simulink model "output_feedback_fixed"  (R2018b)
settings: Solver=VariableStepAuto  StartTime=0.0  StopTime=10  RelTol=1e-3
undefined symbols (not defined in the file): sigbuilder_block
libraries: simulink x1
settings Model: Creator=harkib  LastModifiedBy=Freddy.Kooliyath
settings DebuggingCC: LibraryContextMissingDiagnostic=none
settings SFSimCC: SimUseLocalCustomCode=off
settings RTWCC: RTWUseLocalCustomCode=off

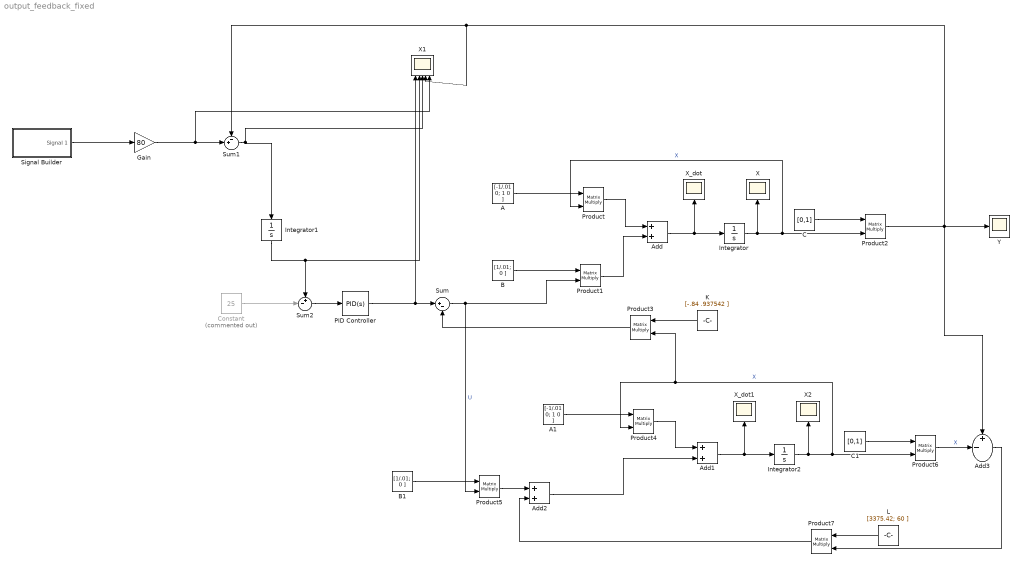
== system output_feedback_fixed ==
  A : Constant  Value=[-1/.01 0; 1 0 ]  VectorParams1D=off
  A1 : Constant  Value=[-1/.01 0; 1 0 ]  VectorParams1D=off
  Add : Sum
  Add1 : Sum
  Add2 : Sum
  Add3 : Sum  Inputs=+-|
  B : Constant  Value=[1/.01; 0 ]  VectorParams1D=off
  B1 : Constant  Value=[1/.01; 0 ]  VectorParams1D=off
  C : Constant  Value=[0,1]  VectorParams1D=off
  C1 : Constant  Value=[0,1]  VectorParams1D=off
  Constant : Constant  Commented=on  Value=25
  Gain : Gain  Gain=80
  Integrator : Integrator
  Integrator1 : Integrator
  Integrator2 : Integrator
  K : Constant  Value=[-.84 .937542 ]  VectorParams1D=off
  L : Constant  Value=[3375.42; 60 ]  VectorParams1D=off
  PID Controller : simulink/Continuous/PID Controller  Controller=PID  Form=Parallel  TimeDomain=Continuous-time  SampleTime=-1  IntegratorMethod=Forward Euler  FilterMethod=Forward Euler  ControllerParametersSource=internal  P=10.0278874654845  I=1.25331489824658  D=2.58452090748358  UseFilter=on  N=1688.62078738213  TunerSelectOption=Transfer Function Based (PID Tuner App)  InitialConditionSource=internal  InitialConditionForIntegrator=0  InitialConditionForFilter=0  DifferentiatorICPrevScaledInput=0  ExternalReset=none  TrackingMode=off  Kt=1  LimitOutput=on  UpperSaturationLimit=inf  LowerSaturationLimit=0  LinearizeAsGain=on  AntiWindupMode=none  Kb=1  POutMin=[]  POutMax=[]  IOutMin=[]  IOutMax=[]  DOutMin=[]  DOutMax=[]  NOutMin=[]  NOutMax=[]  SumOutMin=[]  SumOutMax=[]  SaturationOutMin=[]  SaturationOutMax=[]  PParamMin=[]  PParamMax=[]  IParamMin=[]  IParamMax=[]  DParamMin=[]  DParamMax=[]  NParamMin=[]  NParamMax=[]  KbParamMin=[]  KbParamMax=[]  KtParamMin=[]  KtParamMax=[]  KbOutMin=[]  KbOutMax=[]  KtOutMin=[]  KtOutMax=[]  IntegratorOutMin=[]  IntegratorOutMax=[]  FilterOutMin=[]  FilterOutMax=[]  SumI1OutMin=[]  SumI1OutMax=[]  SumI2OutMin=[]  SumI2OutMax=[]  SumI3OutMin=[]  SumI3OutMax=[]  SumI4OutMin=[]  SumI4OutMax=[]  SumDOutMin=[]  SumDOutMax=[]  DifferentiatorOutMin=[]  DifferentiatorOutMax=[]  FilterDiffOutCoefMin=[]  FilterDiffOutCoefMax=[]  ReciprocalOutMin=[]  ReciprocalOutMax=[]  SumDenOutMin=[]  SumDenOutMax=[]  SumNumOutMin=[]  SumNumOutMax=[]  DivideOutMin=[]  DivideOutMax=[]  IntegratorContinuousStateAttributes=''  IntegratorStateMustResolveToSignalObject=off  IntegratorRTWStateStorageClass=Auto  FilterContinuousStateAttributes=''  FilterStateMustResolveToSignalObject=off  FilterRTWStateStorageClass=Auto  ParallelPVariant=InternalParameters  IdealPVariant=Disabled  IVariant=InternalParameters  DVariant=InternalParameters  IntegratorVariant=Continuous  SatVariant=Enabled  AWVariant=Passthrough  PCopyVariant=Disabled  TRVariant=Disabled  FdbkBlocksVariant=Forward  IdealPFdbkVariant=Disabled  SatFdbkVariant=Disabled  DerivativeFilterVariant=ContFilter  NVariant=InternalParameters  NCopyVariant=Disabled  FilterICVariant=InternalICsFilter  IntegratorICVariant=InternalICs  ExternalResetVariant=Disabled  TRSumVariant=Passthrough  SumFdbkVariant=Disabled  SumVariant=Sum_PID
  Product{,1..7} (8 alike) : Product  Multiplication=Matrix(*)
  Signal Builder : Subsystem  Tag=STV Subsys  LoadFcn=sigbuilder_block('load');  StartFcn=sigbuilder_block('start');  StopFcn=sigbuilder_block('stop');  ClipboardFcn=sigbuilder_block('clipboard');  mask(Sigbuilder block){tuvar=[0:10]}
      mask help: Simulink:masks:SigbuilderBlock_MD
      mask init:
      | if ~strcmp(get_param(bdroot(gcbh),'SimulationStatus'),'stopped') tuvar = sigbuilder_block('maskInit'); end
      settings: CopyFcn=sigbuilder_block('copy');  DeleteFcn=sigbuilder_block('delete');  ModelCloseFcn=sigbuilder_block('modelClose');  PreSaveFcn=sigbuilder_block('preSave');  PauseFcn=sigbuilder_block('pause');  ContinueFcn=sigbuilder_block('continue');  NameChangeFcn=sigbuilder_block('namechange');  OpenFcn=sigbuilder_block('open',[431.25 156 550.5 399.75 ]);  CloseFcn=sigbuilder_block('close');
      mask Display: plot(0, 0, 100, 100,[2, 2, 32, 32, 2], [68, 8, 8, 68, 68],[32, 2], [38, 38], [32, 19, 2],[53, 60, 44], [32, 17, 17, 2],[16, 16, 31, 31]);txt = getActiveGroup(gcbh);text(2, 100, txt,'verticalAlignment', 'top');
  Sum : Sum  Inputs=|+-
  Sum1 : Sum  Inputs=-+|
  Sum2 : Sum  Inputs=+-|
  X : Scope
  X1 : Scope  NumInputPorts=5
  X2 : Scope
  X_dot : Scope
  X_dot1 : Scope
  Y : Scope
  wires:
  Add/1 -> X_dot/1, Integrator/1
  Product1/1 -> Add/2
  Product/1 -> Add/1
  B/1 -> Product1/1
  A/1 -> Product/1
  PID Controller/1 -> X1/1, Sum/1
  K/1 -> Product3/1
  Integrator/1 -> Product2/2, Product/2, X/1  "X"
  Product3/1 -> Sum/2
  Sum/1 -> Product5/2, Product1/2  "U"
  C/1 -> Product2/1
  Product2/1 -> Add3/1, X1/4, Sum1/1, Y/1
  Sum1/1 -> Integrator1/1, X1/3
  Integrator1/1 -> Sum2/1, X1/2
  Gain/1 -> X1/5, Sum1/2
  Signal Builder/1(Signal 1) -> Gain/1
  Sum2/1 -> PID Controller/1
  Constant/1 -> Sum2/2
  Add1/1 -> X_dot1/1, Integrator2/1
  Product4/1 -> Add1/1
  Integrator2/1 -> Product6/2, Product3/2, Product4/2, X2/1  "X"
  C1/1 -> Product6/1
  A1/1 -> Product4/1
  Add2/1 -> Add1/2
  B1/1 -> Product5/1
  Product5/1 -> Add2/1
  L/1 -> Product7/1
  Product7/1 -> Add2/2
  Product6/1 -> Add3/2  "X"
  Add3/1 -> Product7/2

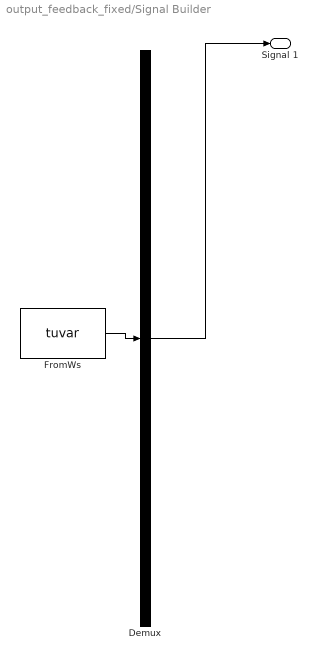
== system output_feedback_fixed/Signal Builder ==
  Demux : Demux  Tag=STV Demux  Outputs=1
  FromWs : FromWorkspace  Tag=STV FromWs  VariableName=tuvar  SampleTime=0
      SigBuilderData=|
      | common.afterFinalStr = 'Extrapolate'
      | common.sampleTime = 0
      | dataSet.timeRange = [0 10]
      | dataSet.name = 'Group 1'
      | sbobj.Groups.Name = 'Group 1'
      | sbobj.Groups.Signals.Name = 'Signal 1'
      | sbobj.Groups.Signals.XData = [0 4 4 6 6 10]
      | sbobj.Groups.Signals.YData = [-0.01 0.005 1 1 0 0]
  Signal 1 : Outport  Tag=STV Outport
  wires:
  Demux/1 -> Signal 1/1
  FromWs/1 -> Demux/1
